simulink model "unity_simu_test"  (R2021b)
settings: Solver=VariableStepAuto  StartTime=0.0  StopTime=10.0  RelTol=1e-3
settings Model: Creator=Duy  LastModifiedBy=Duy

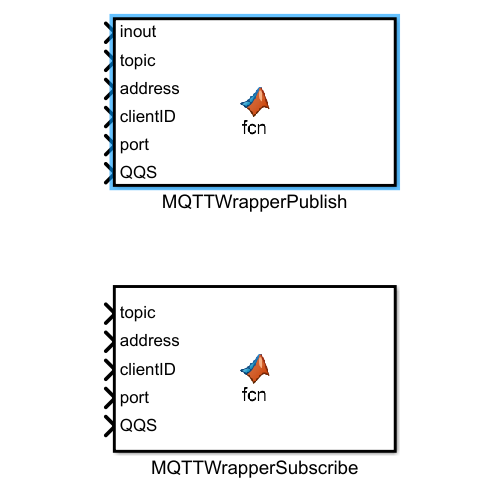
[thumbnail: Simulink's stored preview of the top-level diagram]
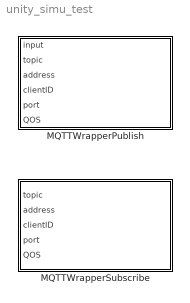
== system unity_simu_test ==
  MQTTWrapperPublish : MATLAB Function  TreatAsAtomicUnit=on
  MQTTWrapperSubscribe : MATLAB Function  TreatAsAtomicUnit=on

== matlab function unity_simu_test/MQTTWrapperPublish ==
  data: input input; topic input; address input; clientID input; port input; QOS input
function fcn(input, topic, address, clientID, port, QOS)
coder.extrinsic('MQTTWrapperPublish')
MQTTWrapperPublish(input, topic, address, clientID, port, QOS)
end

== matlab function unity_simu_test/MQTTWrapperSubscribe ==
  data: topic input; address input; clientID input; port input; QOS input
function fcn(topic, address, clientID, port, QOS)
coder.extrinsic('MQTTWrapperSubscribe')
MQTTWrapperSubscribe(topic, address, clientID, port, QOS)
end
